simulink model "Active_Suspention_v3"  (R2020b)
settings: Solver=VariableStepAuto  StartTime=0.0  StopTime=1  RelTol=1e-3
values from neighbouring files (symbols this model uses):
  Cs = 350    [Suspention.m]
  Ct = 15020    [Suspention.m]
  dynamc_def_factor = 0.4    [Suspention.m]
  Ks = 80000    [Suspention.m]
  Kt = 500000    [Suspention.m]
  Ms = 2500    [Suspention.m]
  Mu = 320    [Suspention.m]
  sprung_acc_factor = 0.3    [Suspention.m]
  travel_sus_factor = 0.3    [Suspention.m]
libraries: dspstat3 x3
settings Model: Creator=sasad  LastModifiedBy=sasad

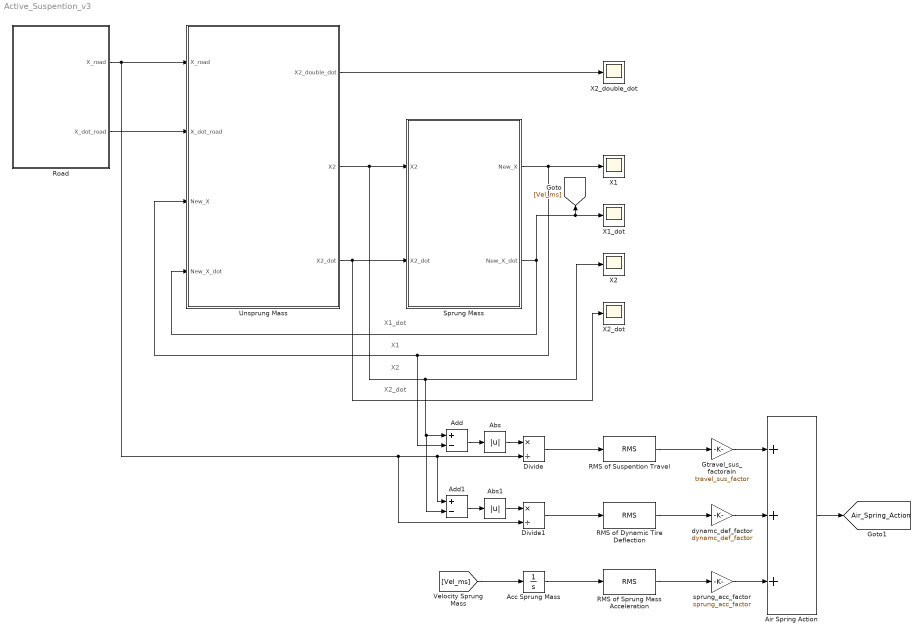
== system Active_Suspention_v3 ==
  note: X1
  note: X2
  note: X1_dot
  note: X2_dot
  Abs : Abs
  Abs1 : Abs
  Acc Sprung Mass : Integrator
  Add : Sum  Inputs=+-
  Add1 : Sum  Inputs=+-
  Air Spring Action : Sum  Inputs=+++
  Divide : Product  Inputs=*/
  Divide1 : Product  Inputs=*/
  Gtravel_sus_factorain : Gain  Gain=travel_sus_factor
  RMS of Dynamic Tire Deflection : dspstat3/RMS  run=off  directionMode=Entire input  dimension=1  InputProcessing=Columns as channels (frame based)  reset_popup=None
  RMS of Sprung Mass Acceleration : dspstat3/RMS  run=off  directionMode=Entire input  dimension=1  InputProcessing=Columns as channels (frame based)  reset_popup=None
  RMS of Suspention Travel : dspstat3/RMS  run=off  directionMode=Entire input  dimension=1  InputProcessing=Columns as channels (frame based)  reset_popup=None
  Road : Subsystem
  Sprung Mass : Subsystem
  Unsprung Mass : Subsystem
  X1 : Scope
  X1_dot : Scope
  X2 : Scope
  X2_dot : Scope
  X2_double_dot : Scope
  dynamc_def_factor : Gain  Gain=dynamc_def_factor
  sprung_acc_factor : Gain  Gain=sprung_acc_factor
  tag scope: Air_Spring_Action=global
  wires:
  Unsprung Mass/2(X2) -> X2/1, Add1/2, Add/1, Sprung Mass/1(X2)
  Unsprung Mass/3(X2_dot) -> X2_dot/1, Sprung Mass/2(X2_dot)
  Sprung Mass/2(New_X_dot) -> Unsprung Mass/4(New_X_dot), [Vel_ms], X1_dot/1
  Sprung Mass/1(New_X) -> X1/1, Add/2, Unsprung Mass/3(New_X)
  Road/1(X_road) -> Divide1/2, Add1/1, Divide/2, Unsprung Mass/1(X_road)
  Road/2(X_dot_road) -> Unsprung Mass/2(X_dot_road)
  Unsprung Mass/1(X2_double_dot) -> X2_double_dot/1
  Add/1 -> Abs/1
  Abs/1 -> Divide/1
  Divide/1 -> RMS of Suspention Travel/1
  Acc Sprung Mass/1 -> RMS of Sprung Mass Acceleration/1
  Abs1/1 -> Divide1/1
  Add1/1 -> Abs1/1
  Divide1/1 -> RMS of Dynamic Tire Deflection/1
  [Vel_ms] -> Acc Sprung Mass/1
  RMS of Dynamic Tire Deflection/1 -> dynamc_def_factor/1
  RMS of Suspention Travel/1 -> Gtravel_sus_factorain/1
  RMS of Sprung Mass Acceleration/1 -> sprung_acc_factor/1
  Gtravel_sus_factorain/1 -> Air Spring Action/1
  dynamc_def_factor/1 -> Air Spring Action/2
  sprung_acc_factor/1 -> Air Spring Action/3
  Air Spring Action/1 -> [Air_Spring_Action]

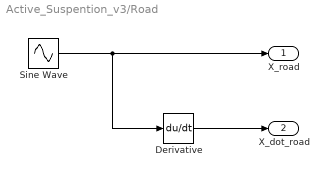
== system Active_Suspention_v3/Road ==
  Derivative : Derivative
  Sine Wave : Sin  Amplitude=0.02  Bias=1  Frequency=0.05  SampleTime=0
  X_road : Outport
  X_dot_road : Outport  Port=2
  wires:
  Derivative/1 -> X_dot_road/1
  Sine Wave/1 -> X_road/1, Derivative/1

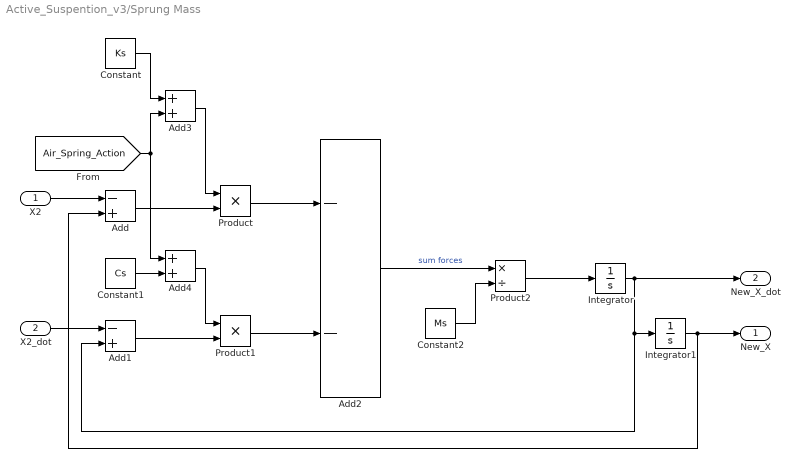
== system Active_Suspention_v3/Sprung Mass ==
  X2 : Inport
  X2_dot : Inport  Port=2
  Add : Sum  Inputs=-+
  Add1 : Sum  Inputs=-+
  Add2 : Sum  Inputs=--
  Add3 : Sum
  Add4 : Sum
  Constant : Constant  Value=Ks
  Constant1 : Constant  Value=Cs
  Constant2 : Constant  Value=Ms
  Integrator : Integrator
  Integrator1 : Integrator
  Product : Product
  Product1 : Product
  Product2 : Product  Inputs=*/
  New_X : Outport
  New_X_dot : Outport  Port=2
  wires:
  Add/1 -> Product/2
  X2_dot/1 -> Add1/1
  X2/1 -> Add/1
  Integrator1/1 -> New_X/1, Add/2
  Add1/1 -> Product1/2
  Product/1 -> Add2/1
  Integrator/1 -> New_X_dot/1, Add1/2, Integrator1/1
  Add2/1 -> Product2/1  "sum forces"
  Product1/1 -> Add2/2
  Product2/1 -> Integrator/1
  Constant2/1 -> Product2/2
  Constant/1 -> Add3/1
  [Air_Spring_Action] -> Add3/2, Add4/1
  Add3/1 -> Product/1
  Constant1/1 -> Add4/2
  Add4/1 -> Product1/1

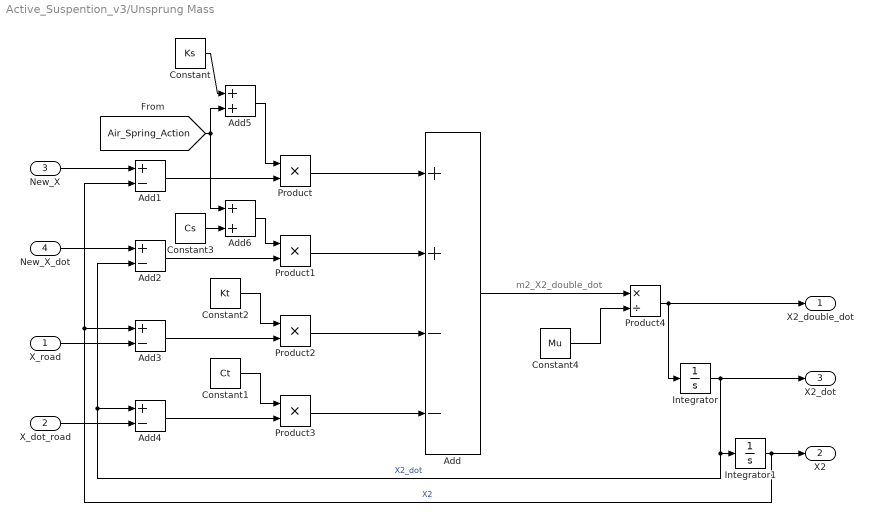
== system Active_Suspention_v3/Unsprung Mass ==
  note: m2_X2_double_dot
  X_road : Inport
  X_dot_road : Inport  Port=2
  New_X : Inport  Port=3
  New_X_dot : Inport  Port=4
  Add : Sum  Inputs=++--
  Add{1..4} (4 alike) : Sum  Inputs=+-
  Add5 : Sum
  Add6 : Sum
  Constant : Constant  Value=Ks
  Constant1 : Constant  Value=Ct
  Constant2 : Constant  Value=Kt
  Constant3 : Constant  Value=Cs
  Constant4 : Constant  Value=Mu
  Integrator : Integrator
  Integrator1 : Integrator
  Product{,1..3} (4 alike) : Product
  Product4 : Product  Inputs=*/
  X2_double_dot : Outport
  X2 : Outport  Port=2
  X2_dot : Outport  Port=3
  wires:
  Integrator1/1 -> X2/1, Add1/2, Add3/1  "X2"
  Integrator/1 -> X2_dot/1, Add2/2, Add4/1, Integrator1/1  "X2_dot"
  Product/1 -> Add/1
  Product2/1 -> Add/3
  Add/1 -> Product4/1
  Constant1/1 -> Product3/1
  Product3/1 -> Add/4
  New_X_dot/1 -> Add2/1
  New_X/1 -> Add1/1
  Add1/1 -> Product/2
  X_road/1 -> Add3/2
  Add4/1 -> Product3/2
  Add3/1 -> Product2/2
  Constant4/1 -> Product4/2
  Product4/1 -> X2_double_dot/1, Integrator/1
  Constant2/1 -> Product2/1
  Product1/1 -> Add/2
  Add2/1 -> Product1/2
  X_dot_road/1 -> Add4/2
  Constant/1 -> Add5/1
  [Air_Spring_Action] -> Add6/1, Add5/2
  Add5/1 -> Product/1
  Constant3/1 -> Add6/2
  Add6/1 -> Product1/1
